simulink model "Pendulo_IvanCalvoSantos"  (R2025b)
settings: Solver=VariableStepAuto  StartTime=0.0  StopTime=10.0  RelTol=1e-3
undefined symbols (not defined in the file): linsys1, linsys2
libraries: nesl_utility x6, fl_lib x2
settings Model: Creator=chenfu  LastModifiedBy=chenfu

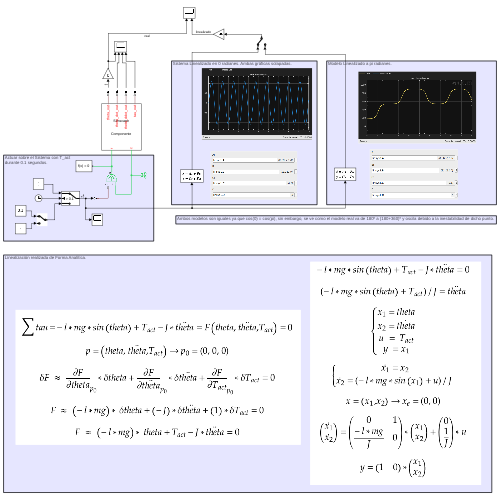
[thumbnail: Simulink's stored preview of the top-level diagram]
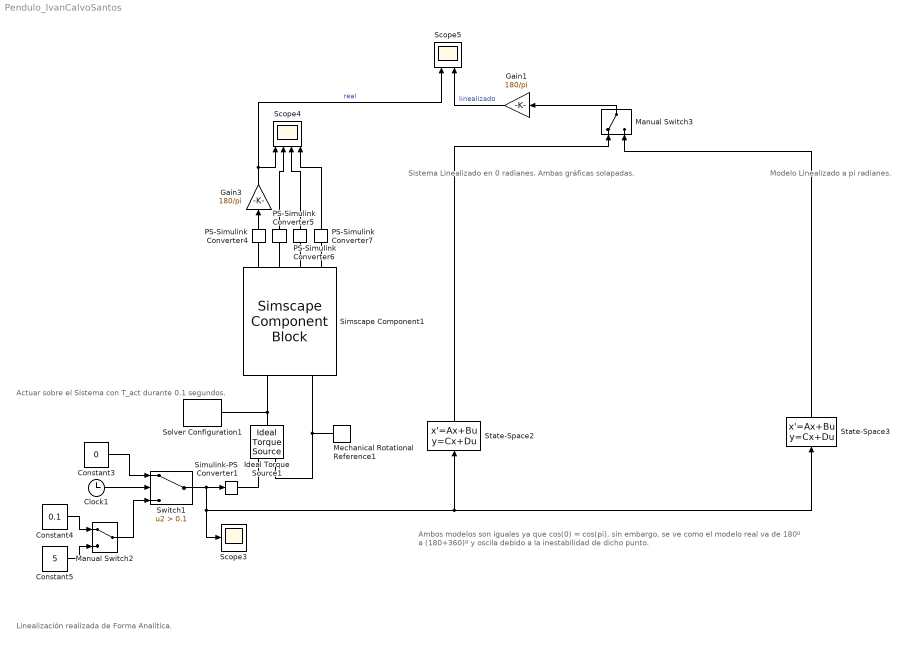
== system Pendulo_IvanCalvoSantos ==
  note: Ambos modelos son iguales ya que cos(0) = cos(pi), sin embargo, se ve como el modelo real va de 180º a (180+360)º y oscila debido a la inestabilidad de dicho punto.
  note: Modelo Linealizado a pi radianes.
  note: Sistema Linealizado en 0 radianes. Ambas gráficas solapadas.
  note: Actuar sobre el Sistema con T_act
      | durante 0.1 segundos.
  note: Linealización realizada de Forma Analítica.
  Clock1 : Clock
  Constant3 : Constant  Value=0
  Constant4 : Constant  Value=0.1
  Constant5 : Constant  Value=5
  Gain1 : Gain  Gain=180/pi
  Gain3 : Gain  Gain=180/pi
  Ideal Torque Source1 : fl_lib/Mechanical/Mechanical Sources/Ideal Torque Source
  Manual Switch2 : ManualSwitch
  Manual Switch3 : ManualSwitch
  Mechanical Rotational Reference1 : fl_lib/Mechanical/Rotational Elements/Mechanical Rotational Reference
  PS-Simulink Converter{4..7} (4 alike) : nesl_utility/PS-Simulink Converter  PhysicalDomain=network_engine_domain  SubClassName=ps_output  LeftPortType=input  RightPortType=output  PseudoPeriodic=off  Frequencies=[]  VectorFormat=inherit  Unit=inherit  AffineConversion=off
  Scope3 : Scope
      settings: ActiveDisplayYMinimum=-1  ActiveDisplayYMaximum=1  DataLoggingVariableName=ScopeData3
  Scope4 : Scope  NumInputPorts=4
      settings: ActiveDisplayYMinimum=-218.42886814795145  ActiveDisplayYMaximum=224.26987423866146  DataLoggingVariableName=ScopeData4
  Scope5 : Scope  NumInputPorts=2
      settings: ActiveDisplayYMinimum=-173.10988777085379  ActiveDisplayYMaximum=1129.9917965122536  DataLoggingVariableName=ScopeData5
  Simscape Component1 : SimscapeComponentBlock  SourceFile=Componente  ComponentPath=Componente  ComponentVariants="[\"Componente\"]"  ComponentVariantNames="[\"Componente\"]"  ClassName=Componente  SchemaVersion=1  m=1 kg  l=0.30 m  g=9.81 m/s^2  w_specify=off  w_priority=High  w=pi rad/s  w_nominal_specify=off  w_nominal_value=1  w_nominal_unit=rad/s  theta_specify=on  theta_priority=None  theta=0 rad  theta_nominal_specify=off  theta_nominal_value=1  theta_nominal_unit=rad  tau_specify=off  tau_priority=None  tau=0 N*m  tau_nominal_specify=off  tau_nominal_value=1  tau_nominal_unit=N*m
      settings: CopyFcn=simscape.sscblock.internal.componentBlockCallback(gcbh,'COPY')  PreCopyFcn=simscape.sscblock.internal.componentBlockCallback(gcbh,'PRECOPY')  PreDeleteFcn=simscape.sscblock.internal.componentBlockCallback(gcbh,'PREDELETE')  InternalSimscapePortConfiguration="{\"Bottom\":[],\"Left\":[{\"id\":\"r\",\"label\":\"r\",\"type\":\"foundation.mechanical.rotational.rotational\"},{\"id\":\"c\",\"label\":\"c\",\"type\":\"foundation.mechanical.rotational.rotational\"}],\"Right\":[{\"id\":\"theta_out\",\"label\":\"theta_out\",\"type\":\"output\"},{\"id\":\"theta_dot_out\",\"label\":\"theta_dot_out\",\"type\":\"output\"},{\"id\":\"theta_ddot_out\",\"label\":\"theta_ddot_out\",\"type\":\"output\"},{\"id\":\"tau_out\",\"label\":\"tau_out\",\"type\":\"output\"}],\"Top\":[]}"
      mask Type: Simple Simscape component
  Simulink-PS Converter1 : nesl_utility/Simulink-PS Converter  PhysicalDomain=network_engine_domain  SubClassName=ps_input  LeftPortType=input  RightPortType=output  PseudoPeriodic=off  Frequencies=[]  NoiseDistribution=none  NoiseParameters=[]  Unit=1  AffineConversion=off  FilteringAndDerivatives=provide  SimscapeFilterOrder=1  InputFilterTimeConstant=0.001  UdotUserProvided=0
  Solver Configuration1 : nesl_utility/Solver Configuration  PhysicalDomain=network_engine_domain  SubClassName=solver  LeftPortType=input  RightPortType=generic  Tones=[]  Harmonics=[]  SimulateNoise=off  Profile=off  UseLocalSampling=off  EnableSwitchedLinearOptims=on  FrequencyDomain=off  UseCCode=off  RelTol=0.001  AbsTol=0.001  MinStep=1e-09  ToWorkspace=off  RevertToSquareIcSolve=off  NumHomotopyIterations=100  PhasorMode=off  PhasorModeNumHarmonics=1  ConsistencySolver=NEWTON_XTOL_AFTER_FTOL  IndexReductionMethod=DerivativeReplacement  DoDC=off  ResidualTolerance=1e-09  ConsistencyTolSource=GLOBAL  ConsistencyAbsTol=0.001  ConsistencyRelTol=0.001  ConsistencyTolFactor=0.001  UseLocalSolver=off  LocalSolverChoice=NE_BACKWARD_EULER_ADVANCER  ResolveIndetEquations=on  FunctionEvalNumThread=1  LocalSolverSampleTime=0.001  DoFixedCost=off  MaxNonlinIter=3  MaxModeIter=2  ComputeImpulses=off  ImpulseIterations=2  LinearAlgebra=auto  LinearAlgebraNumThread=0  EquationFormulation=NE_TIME_EF  DelaysMemoryBudget=1024  AutomaticFiltering=on  FilteringTimeConstant=0.001  PartitionStorageMethod=AS_NEEDED  PartitionMemoryBudget=1024  PartitionMethod=ROBUST  MultibodyUseLocalSolver=off  MultibodyLocalSolverChoice=ODE1  MultibodyLocalSolverSampleTime=0.001
  State-Space2 : StateSpace  A=linsys1.A  B=linsys1.B  C=linsys1.C  D=linsys1.D  InitialCondition=0
  State-Space3 : StateSpace  A=linsys2.A  B=linsys2.B  C=linsys1.C  D=linsys1.D  InitialCondition=0
  Switch1 : Switch  Criteria=u2 > Threshold  Threshold=0.1  SaturateOnIntegerOverflow=off  InputSameDT=off
  wires:
  Switch1/1 -> State-Space2/1, State-Space3/1, Scope3/1, Simulink-PS Converter1/1
  Constant4/1 -> Manual Switch2/1
  Constant5/1 -> Manual Switch2/2
  Manual Switch2/1 -> Switch1/3
  Constant3/1 -> Switch1/1
  Clock1/1 -> Switch1/2
  PS-Simulink Converter5/1 -> Scope4/2
  PS-Simulink Converter4/1 -> Gain3/1
  PS-Simulink Converter6/1 -> Scope4/3
  PS-Simulink Converter7/1 -> Scope4/4
  Gain3/1 -> Scope4/1, Scope5/1  "real"
  State-Space2/1 -> Manual Switch3/1
  State-Space3/1 -> Manual Switch3/2
  Manual Switch3/1 -> Gain1/1
  Gain1/1 -> Scope5/2  "linealizado"
  connections:
  Ideal Torque Source1/LConn1 -- Solver Configuration1/RConn1 -- Simscape Component1/LConn1
  Ideal Torque Source1/RConn2 -- Mechanical Rotational Reference1/LConn1 -- Simscape Component1/LConn2
  Simulink-PS Converter1/RConn1 -- Ideal Torque Source1/RConn1
  Simscape Component1/RConn1 -- PS-Simulink Converter4/LConn1
  Simscape Component1/RConn2 -- PS-Simulink Converter5/LConn1
  Simscape Component1/RConn3 -- PS-Simulink Converter6/LConn1
  Simscape Component1/RConn4 -- PS-Simulink Converter7/LConn1
